simulink model "Model_MS"  (R2018b)
settings: Solver=VariableStepAuto  StartTime=0.0  StopTime=50  MaxStep=1/(100*fn)  MinStep=1/(1000*fn)  RelTol=1e-3
values from neighbouring files (symbols this model uses):
  A = sqrt(2/3)*[1 -0.5 -0.5; 0 sqrt(3)/2 -sqrt(3)/2; sqrt(0.5) sqrt(0.5) sqrt(0.5)]    [Comm_Vect.m]    (also in clarke_conc.m)
  Ai = inv(A)    [Comm_Vect.m]    (also in clarke_conc.m)
  fn = 50    [Comm_Vect.m]    (also in clarke_conc.m)
  fv = 0.0033    [Comm_Vect.m]    (also in clarke_conc.m)
  J = 0.05    [Comm_Vect.m]    (also in clarke_conc.m)
  Ld = 0.245    [Comm_Vect.m]    (also in clarke_conc.m)
  Lq = 0.245    [Comm_Vect.m]    (also in clarke_conc.m)
  p = 60*fn/Nn    (= 2)    [Comm_Vect.m]    (also in clarke_conc.m)
  phi_f = 0.711    [Comm_Vect.m]    (also in clarke_conc.m)
  Rs = 10.5    [Comm_Vect.m]    (also in clarke_conc.m)
  Vn = 220    [Comm_Vect.m]    (also in clarke_conc.m)
  wn = 2*pi*fn    (= 314.159265359)    [Comm_Vect.m]    (also in clarke_conc.m)
undefined symbols (not defined in the file or in its folder): jsin
settings Model: Creator=cindyiskandar  LastModifiedBy=cindyiskandar

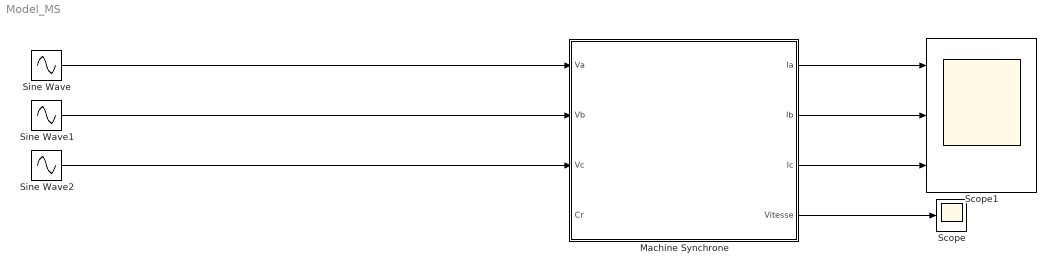
== system Model_MS ==
  Machine Synchrone : Subsystem
  Scope : Scope
  Scope1 : Scope  NumInputPorts=3
  Sine Wave : Sin  Amplitude=Vn  Frequency=2*pi*fn  SampleTime=0
  Sine Wave1 : Sin  Amplitude=Vn  Frequency=2*pi*fn  Phase=2*pi/3  SampleTime=0
  Sine Wave2 : Sin  Amplitude=Vn  Frequency=2*pi*fn  Phase=4*pi/3  SampleTime=0
  wires:
  Sine Wave/1 -> Machine Synchrone/1(Va)
  Sine Wave1/1 -> Machine Synchrone/2(Vb)
  Sine Wave2/1 -> Machine Synchrone/3(Vc)
  Machine Synchrone/1(Ia) -> Scope1/1
  Machine Synchrone/2(Ib) -> Scope1/2
  Machine Synchrone/3(Ic) -> Scope1/3
  Machine Synchrone/4(Vitesse) -> Scope/1

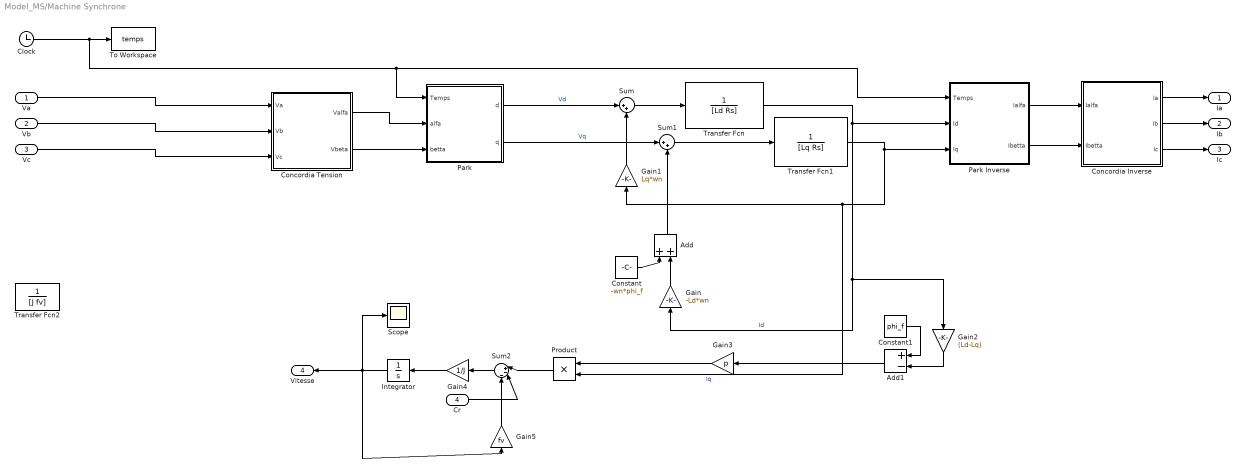
== system Model_MS/Machine Synchrone ==
  Va : Inport
  Vb : Inport  Port=2
  Vc : Inport  Port=3
  Cr : Inport  Port=4
  Add : Sum
  Add1 : Sum  Inputs=+-
  Clock : Clock
  "Concordia Tension " : Subsystem
  "Concordia Inverse " : Subsystem
  Constant : Constant  Value=-wn*phi_f
  Constant1 : Constant  Value=phi_f
  Gain : Gain  Gain=-Ld*wn
  Gain1 : Gain  Gain=Lq*wn
  Gain2 : Gain  Gain=(Ld-Lq)
  Gain3 : Gain  Gain=p
  Gain4 : Gain  Gain=1/J
  Gain5 : Gain  Gain=fv
  Integrator : Integrator
  Park : Subsystem
  Park Inverse : Subsystem
  Product : Product
  Scope : Scope
  Sum : Sum  Inputs=|++
  Sum1 : Sum  Inputs=|++
  Sum2 : Sum  Inputs=|+--
  To Workspace : ToWorkspace  VariableName=temps  SampleTime=-1
      settings: Save2DSignal=2-D array (concatenate along first dimension)
  Transfer Fcn : TransferFcn  Denominator=[Ld Rs]
  Transfer Fcn1 : TransferFcn  Denominator=[Lq Rs]
  Transfer Fcn2 : TransferFcn  Denominator=[J fv]
  Ia : Outport
  Ib : Outport  Port=2
  Ic : Outport  Port=3
  Vitesse : Outport  Port=4
  wires:
  Vb/1 -> "Concordia Tension "/2("Vb ")
  Sum/1 -> Transfer Fcn/1
  Va/1 -> "Concordia Tension "/1("Va ")
  Sum1/1 -> Transfer Fcn1/1
  Product/1 -> Sum2/1
  "Concordia Tension "/2("Vbeta ") -> Park/3("betta ")
  Gain2/1 -> Add1/2
  Gain/1 -> Add/2
  Transfer Fcn1/1 -> Product/2, Gain1/1, Park Inverse/3("Iq ")  "Iq"
  Gain1/1 -> Sum/2
  Vc/1 -> "Concordia Tension "/3(Vc)
  Park/2(q) -> Sum1/1  "Vq"
  Park/1(d) -> Sum/1  "Vd"
  "Concordia Tension "/1(Valfa) -> Park/2(alfa)
  Transfer Fcn/1 -> Gain2/1, Gain/1, Park Inverse/2(Id)  "Id"
  Add/1 -> Sum1/2
  Gain3/1 -> Product/1
  Constant1/1 -> Add1/1
  Add1/1 -> Gain3/1
  Cr/1 -> Sum2/2
  Constant/1 -> Add/1
  Park Inverse/2(Ibetta) -> "Concordia Inverse "/2(Ibetta)
  Park Inverse/1(Ialfa) -> "Concordia Inverse "/1(Ialfa)
  "Concordia Inverse "/1(Ia) -> Ia/1
  "Concordia Inverse "/2(Ib) -> Ib/1
  "Concordia Inverse "/3(Ic) -> Ic/1
  Sum2/1 -> Gain4/1
  Gain5/1 -> Sum2/3
  Gain4/1 -> Integrator/1
  Integrator/1 -> Scope/1, Gain5/1, Vitesse/1
  Clock/1 -> Park Inverse/1("Temps "), Park/1(Temps), To Workspace/1

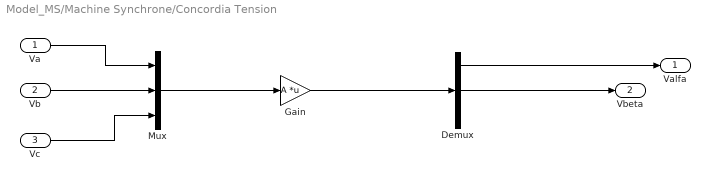
== system Model_MS/Machine Synchrone/Concordia Tension  ==
  "Va " : Inport
  "Vb " : Inport  Port=2
  Vc : Inport  Port=3
  Demux : Demux  Outputs=3
  Gain : Gain  Gain=A  Multiplication=Matrix(K*u) (u vector)
  Mux : Mux  Inputs=3
  Valfa : Outport
  "Vbeta " : Outport  Port=2
  wires:
  Demux/1 -> Valfa/1
  "Va "/1 -> Mux/1
  Mux/1 -> Gain/1
  Gain/1 -> Demux/1
  "Vb "/1 -> Mux/2
  Vc/1 -> Mux/3
  Demux/2 -> "Vbeta "/1

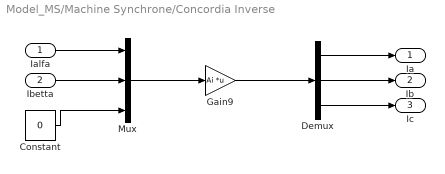
== system Model_MS/Machine Synchrone/Concordia Inverse  ==
  Ialfa : Inport
  Ibetta : Inport  Port=2
  Constant : Constant  Value=0
  Demux : Demux  Outputs=3
  Gain9 : Gain  Gain=Ai  Multiplication=Matrix(K*u) (u vector)
  Mux : Mux  Inputs=3
  Ia : Outport
  Ib : Outport  Port=2
  Ic : Outport  Port=3
  wires:
  Demux/3 -> Ic/1
  Gain9/1 -> Demux/1
  Demux/1 -> Ia/1
  Demux/2 -> Ib/1
  Ibetta/1 -> Mux/2
  Ialfa/1 -> Mux/1
  Mux/1 -> Gain9/1
  Constant/1 -> Mux/3

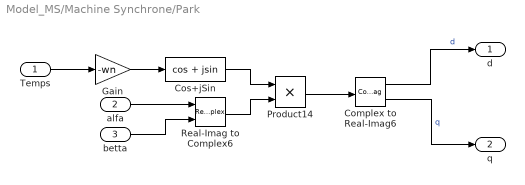
== system Model_MS/Machine Synchrone/Park ==
  Temps : Inport
  alfa : Inport  Port=2
  "betta " : Inport  Port=3
  Complex to Real-Imag6 : ComplexToRealImag
  Cos+jSin : Trigonometry  Operator=cos + jsin
  Gain : Gain  Gain=-wn
  Product14 : Product
  Real-Imag to Complex6 : RealImagToComplex
  d : Outport
  q : Outport  Port=2
  wires:
  alfa/1 -> Real-Imag to Complex6/1
  Product14/1 -> Complex to Real-Imag6/1
  "betta "/1 -> Real-Imag to Complex6/2
  Complex to Real-Imag6/1 -> d/1  "d"
  Complex to Real-Imag6/2 -> q/1  "q"
  Real-Imag to Complex6/1 -> Product14/2
  Cos+jSin/1 -> Product14/1
  Gain/1 -> Cos+jSin/1
  Temps/1 -> Gain/1

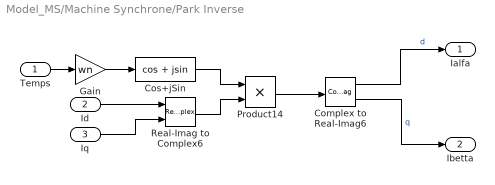
== system Model_MS/Machine Synchrone/Park Inverse ==
  "Temps " : Inport
  Id : Inport  Port=2
  "Iq " : Inport  Port=3
  Complex to Real-Imag6 : ComplexToRealImag
  Cos+jSin : Trigonometry  Operator=cos + jsin
  Gain : Gain  Gain=wn
  Product14 : Product
  Real-Imag to Complex6 : RealImagToComplex
  Ialfa : Outport
  Ibetta : Outport  Port=2
  wires:
  Id/1 -> Real-Imag to Complex6/1
  Product14/1 -> Complex to Real-Imag6/1
  "Iq "/1 -> Real-Imag to Complex6/2
  Complex to Real-Imag6/1 -> Ialfa/1  "d"
  Complex to Real-Imag6/2 -> Ibetta/1  "q"
  Real-Imag to Complex6/1 -> Product14/2
  Cos+jSin/1 -> Product14/1
  Gain/1 -> Cos+jSin/1
  "Temps "/1 -> Gain/1
